simulink model "exampleTutorial"  (R2022a)
settings: Solver=VariableStepAuto  StartTime=0.0  StopTime=10.0  RelTol=1e-3
values from neighbouring files (symbols this model uses):
  b = polyfit(x, y, 1)    [regresion_total.m]    (also in regression_guayas.m = polyfit(a', c', 1))
undefined symbols (not defined in the file or in its folder): k, m, x0
settings Model: Creator=mluser  LastModifiedBy=mluser

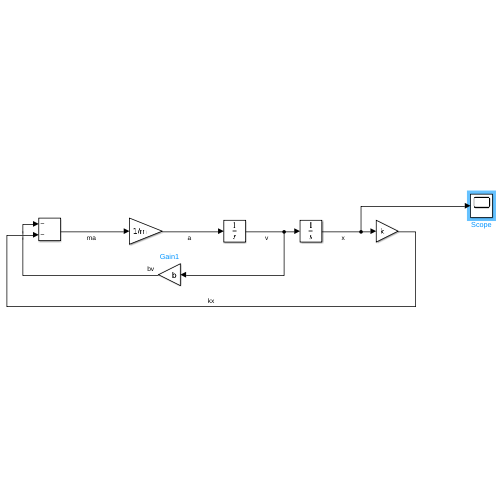
[thumbnail: Simulink's stored preview of the top-level diagram]
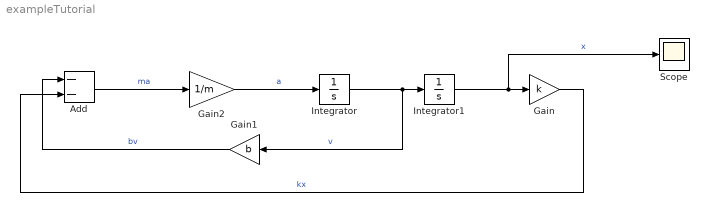
== system exampleTutorial ==
  Add : Sum  Inputs=--
  Gain : Gain  Gain=k
  Gain1 : Gain  Gain=b
  Gain2 : Gain  Gain=1/m
  Integrator : Integrator
  Integrator1 : Integrator  InitialCondition=x0
  Scope : Scope
  wires:
  Gain2/1 -> Integrator/1  "a"
  Integrator/1 -> Gain1/1, Integrator1/1  "v"
  Integrator1/1 -> Gain/1, Scope/1  "x"
  Gain/1 -> Add/2  "kx"
  Gain1/1 -> Add/1  "bv"
  Add/1 -> Gain2/1  "ma"
